simulink model "sdbe_11_11"  (R2012b)
settings: Solver=VariableStepDiscrete  SolverMode=SingleTasking  StartTime=0.0  StopTime=10000  RelTol=1e-3
PreLoadFcn:
  | counter_vals
undefined symbols (not defined in the file or in its folder): sfp
libraries: xbsIndex_r4 x9223, casper_library_misc x39, casper_library_delays x27, dspsigops x16, xps_library x10, r2dbe_vdif_lib x4, r2dbe_adc_lib x3, simulink x1
(part 61 of 78)

== system sdbe_11_11/vdif_2/hdr/w2 ==
  note: 3 bits
  note: According to VDIF documentation for W2
      |
      |
      | bit 31-29 (3): VDIF version number
      | In ALMA EDV it is 0
      |
      | bits 28-24: log2(nchans)
      | 1 channel, so this will be 0
      |
      | bits 23-0: Data Frame length in units
      | of 8 bytes
      | Each 64 bit word is 8 bytes, so 1024 of these
  note: data_fram_length_in_8 byte words
  note: V3
  note: 5 bits
  note: log2(nchans) = 0
  Constant : xbsIndex_r4/Constant  const=0  gui_display_data_type=Fixed-point  arith_type=Unsigned  n_bits=3  bin_pt=0  preci_type=Single  exp_width=8  frac_width=24  explicit_period=on  period=1  equ=P=C  opselect=C  inp2=PCIN>>17  opr=+  inp1=P  carry=CIN  dbl_ovrd=off  block_type=constant
  Constant1 : xbsIndex_r4/Constant  const=3  gui_display_data_type=Fixed-point  arith_type=Unsigned  n_bits=5  bin_pt=0  preci_type=Single  exp_width=8  frac_width=24  explicit_period=on  period=1  equ=P=C  opselect=C  inp2=PCIN>>17  opr=+  inp1=P  carry=CIN  dbl_ovrd=off  block_type=constant
  Constant2 : xbsIndex_r4/Constant  const=132  gui_display_data_type=Fixed-point  arith_type=Unsigned  n_bits=24  bin_pt=0  preci_type=Single  exp_width=8  frac_width=24  explicit_period=on  period=1  equ=P=C  opselect=C  inp2=PCIN>>17  opr=+  inp1=P  carry=CIN  dbl_ovrd=off  block_type=constant
  Convert1 : xbsIndex_r4/Convert  gui_display_data_type=Fixed-point  arith_type=Unsigned  n_bits=32  bin_pt=0  float_type=Single  exp_bits=8  fraction_bits=24  quantization=Truncate  overflow=Wrap  en=off  latency=0  dbl_ovrd=off  pipeline=off  block_type=convert
  Terminator : Terminator
  bus_create : Subsystem  mask(bus_create){inputNum=3}
      mask prompts: inputNum "Number of inputs:"
      mask init:
      | bus_create_init(gcb,...
      |     'inputNum', inputNum);
  frame_len : Subsystem  Tag=xps:sw_reg  AncestorBlock=xps_library/software register  mask(swreg){mode=one value, io_dir=To Processor, io_delay=0, sample_period=1, names=reg, bitwidths=32, arith_types=0, bin_pts=0, sim_port=on, show_format=off}
      mask prompts: io_dir "I/O direction"; io_delay "I/O delay"; sample_period "Sample period"; names "Name:"; bitwidths "Bitwidth:"; arith_types "Type (ufix=0, fix=1, bool=2):"; bin_pts "Binary pt:"; sim_port "Provide sim input/output?"; show_format "Print format string?"
      mask init:
      | swreg_init(gcb)
      settings: AttributesFormatString=1output
      mask TypeOptions mode: one value | fields of equal size | fields of arbitrary size
      mask Callback mode: swreg_cb(gcb);
      mask TypeOptions io_dir: To Processor | From Processor
      mask Callback io_dir:
      | mask_enables = get_param(gcb, 'MaskEnables');
      | mask_names = get_param(gcb, 'MaskNames');
      | if strcmp(get_param(gcb, 'io_dir'), 'To Processor'),
      |     mask_enables{ismember(mask_names, 'sample_period')} = 'off';
      | else
      |     mask_enables{ismember(mask_names, 'sample_period')} = 'on';
      | end
      | set_param(gcb, 'MaskEnables', mask_enables);
      mask Callback bitwidths:
      | swreg_maskcheck(gcb);
      | % blk = gcb;
      | % mode = get_param(blk, 'mode');
      | % current_widths = eval(get_param(blk, 'bitwidths'));
      | % if (strcmp(mode, 'one value') || strcmp(mode, 'fields of equal size')) && (length(current_widths) > 1),
      | %     error('Only one width may be specified for this mode.');
      | % elseif strcmp(mode, 'fields of arbitrary size')
      | %     current_names = textscan(strtrim(strrep(strrep(get_param(blk, 'names'), ']', ''), '[', '')), '%s');
      | %     current_names = current_names{1};
      | %     numios = length(current_names);
      | %     if length(current_widths) ~= numios,
      | %         error('%d field names specified, but %d widths?', numios, length(current_widths));
      | %     end
      | % end
      | % total_width = 0;
      | % for ctr = 1 : length(current_widths),
      | %     total_width = total_width + current_widths(ctr);
      | % end
      | % if total_width > 32,
      | %     error('Total width must be 32 or less, set to %d.', total_width);
      | % end
      mask Callback arith_types:
      | [numios, ~, ~, ~, current_types] = swreg_maskcheck(gcb);
      | % blk = gcb;
      | % mode = get_param(blk, 'mode');
      | % current_types = eval(get_param(blk, 'arith_types'));
      | % numios = length(current_types);
      | % if (strcmp(mode, 'one value') || strcmp(mode, 'fields of equal size')) && (length(current_types) > 1),
      | %     error('Only one type may be specified for this mode.');
      | % elseif strcmp(mode, 'fields of arbitrary size')
      | %     current_names = textscan(strtrim(strrep(strrep(get_param(blk, 'names'), ']', ''), '[', '')), '%s');
      | %     current_names = current_names{1};
      | %     numios = length(current_names);
      | %     if length(current_types) ~= numios,
      | %         error('%d field names specified, but %d types?', numios, length(current_types));
      | %     end
      | % end
      | problem = 0;
      | for ctr = 1 : numios,
      |     t = current_types(ctr);
      |     if (t < 0) || (t > 2),
      |         problem = t;
      |         ctr = numios + 1;
      |     end
      | end
      | if problem ~= 0,
      |     error('Type cannot be %i, must be 0, 1 or 2.', problem);
      | end
      mask Callback bin_pts:
      | swreg_maskcheck(gcb);
      | % blk = gcb;
      | % mode = get_param(blk, 'mode');
      | % current_bins = eval(get_param(blk, 'bin_pts'));
      | % if (strcmp(mode, 'one value') || strcmp(mode, 'fields of equal size')) && (length(current_bins) > 1),
      | %     error('Only one binary pt may be specified for this mode.');
      | % elseif strcmp(mode, 'fields of arbitrary size')
      | %     current_names = textscan(strtrim(strrep(strrep(get_param(blk, 'names'), ']', ''), '[', '')), '%s');
      | %     current_names = current_names{1};
      | %     numios = length(current_names);
      | %     if length(current_bins) ~= numios,
      | %         error('%d field names specified, but %d binary pts?', numios, length(current_bins));
      | %     end
      | % end
  w2 : Outport
  wires:
  Constant1/1 -> bus_create/2(in2)
  bus_create/1(bus_out) -> w2/1
  Constant/1 -> bus_create/1(in1)
  Constant2/1 -> Convert1/1, bus_create/3(in3)
  frame_len/1(sim_out) -> Terminator/1
  Convert1/1 -> frame_len/1(out_reg)

== system sdbe_11_11/vdif_2/hdr/w3 ==
  note: 1 bits
  note: 16 bits
  note: 10 bits
  note: bits per samp minus 1
  note: 5 bits
  note: real_or_comp
  note: According to VDIF documentation for W3
      |
      |
      | bit 31: Real Data or Complex
      | 0 for real data
      |
      | bits 30-26 #bits/sample -1
      | 2 bits per sample -1 =1
      |
      | bits 25-16: thread ID (0 to 1023)
      | not multi-threaded, so just 0
      |
      | Bits 15-0: station ID
  Constant : xbsIndex_r4/Constant  const=1  gui_display_data_type=Fixed-point  arith_type=Unsigned  n_bits=1  bin_pt=0  preci_type=Single  exp_width=8  frac_width=24  explicit_period=on  period=1  equ=P=C  opselect=C  inp2=PCIN>>17  opr=+  inp1=P  carry=CIN  dbl_ovrd=off  block_type=constant
  Constant1 : xbsIndex_r4/Constant  const=1  gui_display_data_type=Fixed-point  arith_type=Unsigned  n_bits=5  bin_pt=0  preci_type=Single  exp_width=8  frac_width=24  explicit_period=on  period=1  equ=P=C  opselect=C  inp2=PCIN>>17  opr=+  inp1=P  carry=CIN  dbl_ovrd=off  block_type=constant
  Constant2 : Constant  Value=1023
  Constant3 : Constant  Value=3097
  Slice : xbsIndex_r4/Slice  nbits=16  boolean_output=off  mode=Lower Bit Location + Width  bit1=0  base1=MSB of Input  bit0=0  base0=LSB of Input  dbl_ovrd=off  block_type=slice
  Slice1 : xbsIndex_r4/Slice  nbits=10  boolean_output=off  mode=Lower Bit Location + Width  bit1=0  base1=MSB of Input  bit0=0  base0=LSB of Input  dbl_ovrd=off  block_type=slice
  bus_create3 : Subsystem  mask(bus_create){inputNum=4}
      mask prompts: inputNum "Number of inputs:"
      mask init:
      | bus_create_init(gcb,...
      |     'inputNum', inputNum);
  pipeline : casper_library_delays/pipeline  latency=1
      settings: AttributesFormatString=Latency = %<latency>
  pipeline1 : casper_library_delays/pipeline  latency=1
      settings: AttributesFormatString=Latency = %<latency>
  station_id : Subsystem  Tag=xps:sw_reg  AncestorBlock=xps_library/software register  mask(swreg){mode=one value, io_dir=From Processor, io_delay=0, sample_period=1, names=reg, bitwidths=32, arith_types=0, bin_pts=0, sim_port=on, show_format=off}
      mask prompts: io_dir "I/O direction"; io_delay "I/O delay"; sample_period "Sample period"; names "Name:"; bitwidths "Bitwidth:"; arith_types "Type (ufix=0, fix=1, bool=2):"; bin_pts "Binary pt:"; sim_port "Provide sim input/output?"; show_format "Print format string?"
      mask init:
      | swreg_init(gcb)
      settings: AttributesFormatString=1input
      mask TypeOptions mode: one value | fields of equal size | fields of arbitrary size
      mask Callback mode: swreg_cb(gcb);
      mask TypeOptions io_dir: To Processor | From Processor
      mask Callback io_dir:
      | mask_enables = get_param(gcb, 'MaskEnables');
      | mask_names = get_param(gcb, 'MaskNames');
      | if strcmp(get_param(gcb, 'io_dir'), 'To Processor'),
      |     mask_enables{ismember(mask_names, 'sample_period')} = 'off';
      | else
      |     mask_enables{ismember(mask_names, 'sample_period')} = 'on';
      | end
      | set_param(gcb, 'MaskEnables', mask_enables);
      mask Callback bitwidths:
      | swreg_maskcheck(gcb);
      | % blk = gcb;
      | % mode = get_param(blk, 'mode');
      | % current_widths = eval(get_param(blk, 'bitwidths'));
      | % if (strcmp(mode, 'one value') || strcmp(mode, 'fields of equal size')) && (length(current_widths) > 1),
      | %     error('Only one width may be specified for this mode.');
      | % elseif strcmp(mode, 'fields of arbitrary size')
      | %     current_names = textscan(strtrim(strrep(strrep(get_param(blk, 'names'), ']', ''), '[', '')), '%s');
      | %     current_names = current_names{1};
      | %     numios = length(current_names);
      | %     if length(current_widths) ~= numios,
      | %         error('%d field names specified, but %d widths?', numios, length(current_widths));
      | %     end
      | % end
      | % total_width = 0;
      | % for ctr = 1 : length(current_widths),
      | %     total_width = total_width + current_widths(ctr);
      | % end
      | % if total_width > 32,
      | %     error('Total width must be 32 or less, set to %d.', total_width);
      | % end
      mask Callback arith_types:
      | [numios, ~, ~, ~, current_types] = swreg_maskcheck(gcb);
      | % blk = gcb;
      | % mode = get_param(blk, 'mode');
      | % current_types = eval(get_param(blk, 'arith_types'));
      | % numios = length(current_types);
      | % if (strcmp(mode, 'one value') || strcmp(mode, 'fields of equal size')) && (length(current_types) > 1),
      | %     error('Only one type may be specified for this mode.');
      | % elseif strcmp(mode, 'fields of arbitrary size')
      | %     current_names = textscan(strtrim(strrep(strrep(get_param(blk, 'names'), ']', ''), '[', '')), '%s');
      | %     current_names = current_names{1};
      | %     numios = length(current_names);
      | %     if length(current_types) ~= numios,
      | %         error('%d field names specified, but %d types?', numios, length(current_types));
      | %     end
      | % end
      | problem = 0;
      | for ctr = 1 : numios,
      |     t = current_types(ctr);
      |     if (t < 0) || (t > 2),
      |         problem = t;
      |         ctr = numios + 1;
      |     end
      | end
      | if problem ~= 0,
      |     error('Type cannot be %i, must be 0, 1 or 2.', problem);
      | end
      mask Callback bin_pts:
      | swreg_maskcheck(gcb);
      | % blk = gcb;
      | % mode = get_param(blk, 'mode');
      | % current_bins = eval(get_param(blk, 'bin_pts'));
      | % if (strcmp(mode, 'one value') || strcmp(mode, 'fields of equal size')) && (length(current_bins) > 1),
      | %     error('Only one binary pt may be specified for this mode.');
      | % elseif strcmp(mode, 'fields of arbitrary size')
      | %     current_names = textscan(strtrim(strrep(strrep(get_param(blk, 'names'), ']', ''), '[', '')), '%s');
      | %     current_names = current_names{1};
      | %     numios = length(current_names);
      | %     if length(current_bins) ~= numios,
      | %         error('%d field names specified, but %d binary pts?', numios, length(current_bins));
      | %     end
      | % end
  thread_id : Subsystem  Tag=xps:sw_reg  AncestorBlock=xps_library/software register  mask(swreg){mode=one value, io_dir=From Processor, io_delay=0, sample_period=1, names=reg, bitwidths=32, arith_types=0, bin_pts=0, sim_port=on, show_format=off}
      mask prompts: io_dir "I/O direction"; io_delay "I/O delay"; sample_period "Sample period"; names "Name:"; bitwidths "Bitwidth:"; arith_types "Type (ufix=0, fix=1, bool=2):"; bin_pts "Binary pt:"; sim_port "Provide sim input/output?"; show_format "Print format string?"
      mask init:
      | swreg_init(gcb)
      settings: AttributesFormatString=1input
      mask TypeOptions mode: one value | fields of equal size | fields of arbitrary size
      mask Callback mode: swreg_cb(gcb);
      mask TypeOptions io_dir: To Processor | From Processor
      mask Callback io_dir:
      | mask_enables = get_param(gcb, 'MaskEnables');
      | mask_names = get_param(gcb, 'MaskNames');
      | if strcmp(get_param(gcb, 'io_dir'), 'To Processor'),
      |     mask_enables{ismember(mask_names, 'sample_period')} = 'off';
      | else
      |     mask_enables{ismember(mask_names, 'sample_period')} = 'on';
      | end
      | set_param(gcb, 'MaskEnables', mask_enables);
      mask Callback bitwidths:
      | swreg_maskcheck(gcb);
      | % blk = gcb;
      | % mode = get_param(blk, 'mode');
      | % current_widths = eval(get_param(blk, 'bitwidths'));
      | % if (strcmp(mode, 'one value') || strcmp(mode, 'fields of equal size')) && (length(current_widths) > 1),
      | %     error('Only one width may be specified for this mode.');
      | % elseif strcmp(mode, 'fields of arbitrary size')
      | %     current_names = textscan(strtrim(strrep(strrep(get_param(blk, 'names'), ']', ''), '[', '')), '%s');
      | %     current_names = current_names{1};
      | %     numios = length(current_names);
      | %     if length(current_widths) ~= numios,
      | %         error('%d field names specified, but %d widths?', numios, length(current_widths));
      | %     end
      | % end
      | % total_width = 0;
      | % for ctr = 1 : length(current_widths),
      | %     total_width = total_width + current_widths(ctr);
      | % end
      | % if total_width > 32,
      | %     error('Total width must be 32 or less, set to %d.', total_width);
      | % end
      mask Callback arith_types:
      | [numios, ~, ~, ~, current_types] = swreg_maskcheck(gcb);
      | % blk = gcb;
      | % mode = get_param(blk, 'mode');
      | % current_types = eval(get_param(blk, 'arith_types'));
      | % numios = length(current_types);
      | % if (strcmp(mode, 'one value') || strcmp(mode, 'fields of equal size')) && (length(current_types) > 1),
      | %     error('Only one type may be specified for this mode.');
      | % elseif strcmp(mode, 'fields of arbitrary size')
      | %     current_names = textscan(strtrim(strrep(strrep(get_param(blk, 'names'), ']', ''), '[', '')), '%s');
      | %     current_names = current_names{1};
      | %     numios = length(current_names);
      | %     if length(current_types) ~= numios,
      | %         error('%d field names specified, but %d types?', numios, length(current_types));
      | %     end
      | % end
      | problem = 0;
      | for ctr = 1 : numios,
      |     t = current_types(ctr);
      |     if (t < 0) || (t > 2),
      |         problem = t;
      |         ctr = numios + 1;
      |     end
      | end
      | if problem ~= 0,
      |     error('Type cannot be %i, must be 0, 1 or 2.', problem);
      | end
      mask Callback bin_pts:
      | swreg_maskcheck(gcb);
      | % blk = gcb;
      | % mode = get_param(blk, 'mode');
      | % current_bins = eval(get_param(blk, 'bin_pts'));
      | % if (strcmp(mode, 'one value') || strcmp(mode, 'fields of equal size')) && (length(current_bins) > 1),
      | %     error('Only one binary pt may be specified for this mode.');
      | % elseif strcmp(mode, 'fields of arbitrary size')
      | %     current_names = textscan(strtrim(strrep(strrep(get_param(blk, 'names'), ']', ''), '[', '')), '%s');
      | %     current_names = current_names{1};
      | %     numios = length(current_names);
      | %     if length(current_bins) ~= numios,
      | %         error('%d field names specified, but %d binary pts?', numios, length(current_bins));
      | %     end
      | % end
  w3 : Outport
  wires:
  pipeline1/1 -> Slice/1
  pipeline/1 -> Slice1/1
  Slice/1 -> bus_create3/4(in4)
  Constant/1 -> bus_create3/1(in1)
  Slice1/1 -> bus_create3/3(in3)
  Constant1/1 -> bus_create3/2(in2)
  thread_id/1(in_reg) -> pipeline/1
  Constant2/1 -> thread_id/1(sim_1)
  Constant3/1 -> station_id/1(sim_1)
  station_id/1(in_reg) -> pipeline1/1
  bus_create3/1(bus_out) -> w3/1

== system sdbe_11_11/vdif_2/hdr/w6_w7 ==
  note: in simulation because I don't have the fixed point tool kit,
      | the 64 bit counter is messing up so I am getting values starting with 1 rather than 0
      | I think in compile this will work
  note: start this at 2^64-1, so its the last value of the counter,
      | then when enabled the first value will be 0
  note: According to VDIF documentation for W5
      | and EDV doc for ALMA
      |
      | not sure what the packet serial number is,
      | apparently it is appended in front of the packet
      | for transfer, but im not sure where it comes from
      |
      | This uses UDP, so I wonder when it is appended
      |
      | Right now I have a software register in there as a place holder
  note: word 7 is MOst sig 32
  note: word 6 is Least sig
  start_of_frame : Inport
  Convert1 : xbsIndex_r4/Convert  gui_display_data_type=Fixed-point  arith_type=Unsigned  n_bits=32  bin_pt=0  float_type=Single  exp_bits=8  fraction_bits=24  quantization=Truncate  overflow=Wrap  en=off  latency=0  dbl_ovrd=off  pipeline=off  block_type=convert
  Convert2 : xbsIndex_r4/Convert  gui_display_data_type=Fixed-point  arith_type=Unsigned  n_bits=32  bin_pt=0  float_type=Single  exp_bits=8  fraction_bits=24  quantization=Truncate  overflow=Wrap  en=off  latency=0  dbl_ovrd=off  pipeline=off  block_type=convert
  Counter : xbsIndex_r4/Counter  cnt_type=Free Running  cnt_to=Inf  operation=Up  start_count=2^64-1  cnt_by_val=1  arith_type=Unsigned  n_bits=64  bin_pt=0  load_pin=off  rst=off  en=on  explicit_period=on  period=1  dbl_ovrd=off  use_behavioral_HDL=off  implementation=Fabric  block_type=counter
  Delay : xbsIndex_r4/Delay  rst=off  infoeditControl=Selection of Reset will increase slice count due to use of real FFs and instead of SRLs  en=off  latency=1  dbl_ovrd=off  reg_retiming=off  block_type=delay
  Delay1 : xbsIndex_r4/Delay  rst=off  infoeditControl=Selection of Reset will increase slice count due to use of real FFs and instead of SRLs  en=off  latency=1  dbl_ovrd=off  reg_retiming=off  block_type=delay
  Terminator : Terminator
  Terminator1 : Terminator
  lower_32 : xbsIndex_r4/Slice  nbits=32  boolean_output=off  mode=Lower Bit Location + Width  bit1=0  base1=LSB of Input  bit0=0  base0=LSB of Input  dbl_ovrd=off  block_type=slice
  psn_high : Subsystem  Tag=xps:sw_reg  AncestorBlock=xps_library/software register  mask(swreg){mode=one value, io_dir=To Processor, io_delay=0, sample_period=1, names=reg, bitwidths=32, arith_types=0, bin_pts=0, sim_port=on, show_format=off}
      mask prompts: io_dir "I/O direction"; io_delay "I/O delay"; sample_period "Sample period"; names "Name:"; bitwidths "Bitwidth:"; arith_types "Type (ufix=0, fix=1, bool=2):"; bin_pts "Binary pt:"; sim_port "Provide sim input/output?"; show_format "Print format string?"
      mask init:
      | swreg_init(gcb)
      settings: AttributesFormatString=1output
      mask TypeOptions mode: one value | fields of equal size | fields of arbitrary size
      mask Callback mode: swreg_cb(gcb);
      mask TypeOptions io_dir: To Processor | From Processor
      mask Callback io_dir:
      | mask_enables = get_param(gcb, 'MaskEnables');
      | mask_names = get_param(gcb, 'MaskNames');
      | if strcmp(get_param(gcb, 'io_dir'), 'To Processor'),
      |     mask_enables{ismember(mask_names, 'sample_period')} = 'off';
      | else
      |     mask_enables{ismember(mask_names, 'sample_period')} = 'on';
      | end
      | set_param(gcb, 'MaskEnables', mask_enables);
      mask Callback bitwidths:
      | swreg_maskcheck(gcb);
      | % blk = gcb;
      | % mode = get_param(blk, 'mode');
      | % current_widths = eval(get_param(blk, 'bitwidths'));
      | % if (strcmp(mode, 'one value') || strcmp(mode, 'fields of equal size')) && (length(current_widths) > 1),
      | %     error('Only one width may be specified for this mode.');
      | % elseif strcmp(mode, 'fields of arbitrary size')
      | %     current_names = textscan(strtrim(strrep(strrep(get_param(blk, 'names'), ']', ''), '[', '')), '%s');
      | %     current_names = current_names{1};
      | %     numios = length(current_names);
      | %     if length(current_widths) ~= numios,
      | %         error('%d field names specified, but %d widths?', numios, length(current_widths));
      | %     end
      | % end
      | % total_width = 0;
      | % for ctr = 1 : length(current_widths),
      | %     total_width = total_width + current_widths(ctr);
      | % end
      | % if total_width > 32,
      | %     error('Total width must be 32 or less, set to %d.', total_width);
      | % end
      mask Callback arith_types:
      | [numios, ~, ~, ~, current_types] = swreg_maskcheck(gcb);
      | % blk = gcb;
      | % mode = get_param(blk, 'mode');
      | % current_types = eval(get_param(blk, 'arith_types'));
      | % numios = length(current_types);
      | % if (strcmp(mode, 'one value') || strcmp(mode, 'fields of equal size')) && (length(current_types) > 1),
      | %     error('Only one type may be specified for this mode.');
      | % elseif strcmp(mode, 'fields of arbitrary size')
      | %     current_names = textscan(strtrim(strrep(strrep(get_param(blk, 'names'), ']', ''), '[', '')), '%s');
      | %     current_names = current_names{1};
      | %     numios = length(current_names);
      | %     if length(current_types) ~= numios,
      | %         error('%d field names specified, but %d types?', numios, length(current_types));
      | %     end
      | % end
      | problem = 0;
      | for ctr = 1 : numios,
      |     t = current_types(ctr);
      |     if (t < 0) || (t > 2),
      |         problem = t;
      |         ctr = numios + 1;
      |     end
      | end
      | if problem ~= 0,
      |     error('Type cannot be %i, must be 0, 1 or 2.', problem);
      | end
      mask Callback bin_pts:
      | swreg_maskcheck(gcb);
      | % blk = gcb;
      | % mode = get_param(blk, 'mode');
      | % current_bins = eval(get_param(blk, 'bin_pts'));
      | % if (strcmp(mode, 'one value') || strcmp(mode, 'fields of equal size')) && (length(current_bins) > 1),
      | %     error('Only one binary pt may be specified for this mode.');
      | % elseif strcmp(mode, 'fields of arbitrary size')
      | %     current_names = textscan(strtrim(strrep(strrep(get_param(blk, 'names'), ']', ''), '[', '')), '%s');
      | %     current_names = current_names{1};
      | %     numios = length(current_names);
      | %     if length(current_bins) ~= numios,
      | %         error('%d field names specified, but %d binary pts?', numios, length(current_bins));
      | %     end
      | % end
  psn_low : Subsystem  Tag=xps:sw_reg  AncestorBlock=xps_library/software register  mask(swreg){mode=one value, io_dir=To Processor, io_delay=0, sample_period=1, names=reg, bitwidths=32, arith_types=0, bin_pts=0, sim_port=on, show_format=off}
      mask prompts: io_dir "I/O direction"; io_delay "I/O delay"; sample_period "Sample period"; names "Name:"; bitwidths "Bitwidth:"; arith_types "Type (ufix=0, fix=1, bool=2):"; bin_pts "Binary pt:"; sim_port "Provide sim input/output?"; show_format "Print format string?"
      mask init:
      | swreg_init(gcb)
      settings: AttributesFormatString=1output
      mask TypeOptions mode: one value | fields of equal size | fields of arbitrary size
      mask Callback mode: swreg_cb(gcb);
      mask TypeOptions io_dir: To Processor | From Processor
      mask Callback io_dir:
      | mask_enables = get_param(gcb, 'MaskEnables');
      | mask_names = get_param(gcb, 'MaskNames');
      | if strcmp(get_param(gcb, 'io_dir'), 'To Processor'),
      |     mask_enables{ismember(mask_names, 'sample_period')} = 'off';
      | else
      |     mask_enables{ismember(mask_names, 'sample_period')} = 'on';
      | end
      | set_param(gcb, 'MaskEnables', mask_enables);
      mask Callback bitwidths:
      | swreg_maskcheck(gcb);
      | % blk = gcb;
      | % mode = get_param(blk, 'mode');
      | % current_widths = eval(get_param(blk, 'bitwidths'));
      | % if (strcmp(mode, 'one value') || strcmp(mode, 'fields of equal size')) && (length(current_widths) > 1),
      | %     error('Only one width may be specified for this mode.');
      | % elseif strcmp(mode, 'fields of arbitrary size')
      | %     current_names = textscan(strtrim(strrep(strrep(get_param(blk, 'names'), ']', ''), '[', '')), '%s');
      | %     current_names = current_names{1};
      | %     numios = length(current_names);
      | %     if length(current_widths) ~= numios,
      | %         error('%d field names specified, but %d widths?', numios, length(current_widths));
      | %     end
      | % end
      | % total_width = 0;
      | % for ctr = 1 : length(current_widths),
      | %     total_width = total_width + current_widths(ctr);
      | % end
      | % if total_width > 32,
      | %     error('Total width must be 32 or less, set to %d.', total_width);
      | % end
      mask Callback arith_types:
      | [numios, ~, ~, ~, current_types] = swreg_maskcheck(gcb);
      | % blk = gcb;
      | % mode = get_param(blk, 'mode');
      | % current_types = eval(get_param(blk, 'arith_types'));
      | % numios = length(current_types);
      | % if (strcmp(mode, 'one value') || strcmp(mode, 'fields of equal size')) && (length(current_types) > 1),
      | %     error('Only one type may be specified for this mode.');
      | % elseif strcmp(mode, 'fields of arbitrary size')
      | %     current_names = textscan(strtrim(strrep(strrep(get_param(blk, 'names'), ']', ''), '[', '')), '%s');
      | %     current_names = current_names{1};
      | %     numios = length(current_names);
      | %     if length(current_types) ~= numios,
      | %         error('%d field names specified, but %d types?', numios, length(current_types));
      | %     end
      | % end
      | problem = 0;
      | for ctr = 1 : numios,
      |     t = current_types(ctr);
      |     if (t < 0) || (t > 2),
      |         problem = t;
      |         ctr = numios + 1;
      |     end
      | end
      | if problem ~= 0,
      |     error('Type cannot be %i, must be 0, 1 or 2.', problem);
      | end
      mask Callback bin_pts:
      | swreg_maskcheck(gcb);
      | % blk = gcb;
      | % mode = get_param(blk, 'mode');
      | % current_bins = eval(get_param(blk, 'bin_pts'));
      | % if (strcmp(mode, 'one value') || strcmp(mode, 'fields of equal size')) && (length(current_bins) > 1),
      | %     error('Only one binary pt may be specified for this mode.');
      | % elseif strcmp(mode, 'fields of arbitrary size')
      | %     current_names = textscan(strtrim(strrep(strrep(get_param(blk, 'names'), ']', ''), '[', '')), '%s');
      | %     current_names = current_names{1};
      | %     numios = length(current_names);
      | %     if length(current_bins) ~= numios,
      | %         error('%d field names specified, but %d binary pts?', numios, length(current_bins));
      | %     end
      | % end
  upper_32 : xbsIndex_r4/Slice  nbits=32  boolean_output=off  mode=Lower Bit Location + Width  bit1=0  base1=MSB of Input  bit0=32  base0=LSB of Input  dbl_ovrd=off  block_type=slice
  w6 : Outport
  w7 : Outport  Port=2
  wires:
  start_of_frame/1 -> Counter/1
  upper_32/1 -> Convert2/1, Delay/1
  lower_32/1 -> Convert1/1, Delay1/1
  Counter/1 -> lower_32/1, upper_32/1
  psn_low/1(sim_out) -> Terminator/1
  Convert1/1 -> psn_low/1(out_reg)
  psn_high/1(sim_out) -> Terminator1/1
  Convert2/1 -> psn_high/1(out_reg)
  Delay/1 -> w7/1
  Delay1/1 -> w6/1

== system sdbe_11_11/vdif_2/hdr_to_scope1/diagnose_beng_hdr ==
  tx_data : Inport
  tx_val : Inport  Port=2
  Disregard Subsystem : xbsIndex_r4/Disregard Subsystem  Tag=discardX  block_type=disregard
  Scope : Scope  NumInputPorts=2
      settings: TimeRange=1.649420126233963  YMin=-1~-1  YMax=1~1
  wires:
  tx_data/1 -> Scope/1  "data"
  tx_val/1 -> Scope/2  "vals"

== system sdbe_11_11/vdif_2/hdr_to_scope3/beng_w45 ==
  note: VTP so need to wait one more clock
  data : Inport
  val : Inport  Port=2
  spec_val : Inport  Port=3
  Constant : xbsIndex_r4/Constant  const=0  gui_display_data_type=Fixed-point  arith_type=Unsigned  n_bits=64  bin_pt=0  preci_type=Single  exp_width=8  frac_width=24  explicit_period=on  period=1  equ=P=C  opselect=C  inp2=PCIN>>17  opr=+  inp1=P  carry=CIN  dbl_ovrd=off  block_type=constant
  Disregard Subsystem : xbsIndex_r4/Disregard Subsystem  Tag=discardX  block_type=disregard
  Gateway Out{,1..4} (5 alike) : xbsIndex_r4/Gateway Out  inherit_from_input=off  hdl_port=on  timing_constraint=None  locs_specified=off  LOCs={}  UseAsDAC=off  DACChannel='1'  block_type=gatewayout
  Mux : xbsIndex_r4/Mux  inputs=2  en=off  latency=0  precision=Full  arith_type=Unsigned  n_bits=16  bin_pt=14  quantization=Truncate  overflow=Wrap  dbl_ovrd=off  block_type=mux
  Mux1 : Mux  Inputs=2
  Mux2 : Mux  Inputs=3
  Scope : Scope  NumInputPorts=2
      settings: TimeRange=1.649420126233963  YMin=-1~-1  YMax=1~1  SaveName=ScopeData14
  beng_hdr_from_data : Subsystem
  wires:
  val/1 -> Gateway Out3/1
  Gateway Out2/1 -> Mux2/3
  Gateway Out/1 -> Mux2/1
  Constant/1 -> Mux/2
  Mux/1 -> beng_hdr_from_data/1(hdr_64)
  [val_45] -> Mux/1
  Mux1/1 -> Scope/2  "val_yellow__w45_val_pink"
  Gateway Out1/1 -> Mux2/2
  beng_hdr_from_data/3(fcount) -> Gateway Out2/1
  Gateway Out3/1 -> Mux1/1
  Gateway Out4/1 -> Mux1/2
  data/1 -> Mux/3
  beng_hdr_from_data/2(bcount) -> Gateway Out1/1
  beng_hdr_from_data/1(ccount) -> Gateway Out/1
  spec_val/1 -> Gateway Out4/1, [val_45]
  Mux2/1 -> Scope/1  "c_yellow__b_pink__f_blue"

== system sdbe_11_11/vdif_2/hdr_to_scope3/data_p0r ==
  note: VTP so need to wait one more clock
  data : Inport
  val : Inport  Port=2
  spec_val : Inport  Port=3
  Constant : xbsIndex_r4/Constant  const=0  gui_display_data_type=Fixed-point  arith_type=Unsigned  n_bits=64  bin_pt=0  preci_type=Single  exp_width=8  frac_width=24  explicit_period=on  period=1  equ=P=C  opselect=C  inp2=PCIN>>17  opr=+  inp1=P  carry=CIN  dbl_ovrd=off  block_type=constant
  Disregard Subsystem : xbsIndex_r4/Disregard Subsystem  Tag=discardX  block_type=disregard
  Gateway Out{1..40} (40 alike) : xbsIndex_r4/Gateway Out  inherit_from_input=off  hdl_port=on  timing_constraint=None  locs_specified=off  LOCs={}  UseAsDAC=off  DACChannel='1'  block_type=gatewayout
  Mux : xbsIndex_r4/Mux  inputs=2  en=off  latency=0  precision=Full  arith_type=Unsigned  n_bits=16  bin_pt=14  quantization=Truncate  overflow=Wrap  dbl_ovrd=off  block_type=mux
  Mux{1,3,5,7} (4 alike) : Mux  Inputs=2
  Mux{2,4,6,8} (4 alike) : Mux  Inputs=8
  Scope{,1..3} (4 alike) : Scope  NumInputPorts=2
      Scope settings: TimeRange=1.649420126233963  YMin=-1~-1  YMax=1~1  SaveName=ScopeData12
      Scope1 settings: TimeRange=1.649420126233963  YMin=-1~-1  YMax=1~1  SaveName=ScopeData18
      Scope2 settings: TimeRange=1.649420126233963  YMin=-1~-1  YMax=1~1  SaveName=ScopeData19
      Scope3 settings: TimeRange=1.649420126233963  YMin=-1~-1  YMax=1~1  SaveName=ScopeData20
  Subsystem : Subsystem
  bus_expand : Subsystem  AncestorBlock=casper_library_flow_control/bus_expand  mask(bus_expand){mode=divisions of equal size, outputNum=8, outputWidth=2, outputBinaryPt=0, outputArithmeticType=0, show_format=off, outputToWorkspace=off, variablePrefix=out, outputToModelAsWell=on}
      mask prompts: outputNum "Number of outputs:"; outputWidth "Output width:"; outputBinaryPt "Output binary point position:"; outputArithmeticType "Output arithmetic type (ufix=0, fix=1, bool=2):"; show_format "Print format string?"; outputToWorkspace "Output to workspace?"; variablePrefix "Variable name prefix:"; outputToModelAsWell "Output to model as well?"
      mask help:
      | Expands a 'bus' made using a bus_create or Xilinx
      | concat block.
      | The input will be divided into the specified number
      | of outputs with the specified arithmetic types.
      | Divisions are made from most significant bit.
      mask init: same as sdbe_11_11/get_data_from_pkt/scope/bus_expand1
      settings: AttributesFormatString=8 outputs
      mask TypeOptions mode: divisions of equal size | divisions of arbitrary size
      mask Callback mode: bus_expand_callback();
      mask Callback outputWidth: bus_expand_callback();
      mask Callback outputToWorkspace: bus_expand_callback();
  bus_expand1 : Subsystem  AncestorBlock=casper_library_flow_control/bus_expand  mask(bus_expand){mode=divisions of equal size, outputNum=8, outputWidth=2, outputBinaryPt=0, outputArithmeticType=0, show_format=off, outputToWorkspace=off, variablePrefix=out, outputToModelAsWell=on}
      mask prompts: outputNum "Number of outputs:"; outputWidth "Output width:"; outputBinaryPt "Output binary point position:"; outputArithmeticType "Output arithmetic type (ufix=0, fix=1, bool=2):"; show_format "Print format string?"; outputToWorkspace "Output to workspace?"; variablePrefix "Variable name prefix:"; outputToModelAsWell "Output to model as well?"
      mask help:
      | Expands a 'bus' made using a bus_create or Xilinx
      | concat block.
      | The input will be divided into the specified number
      | of outputs with the specified arithmetic types.
      | Divisions are made from most significant bit.
      mask init: same as sdbe_11_11/get_data_from_pkt/scope/bus_expand1
      settings: AttributesFormatString=8 outputs
      mask TypeOptions mode: divisions of equal size | divisions of arbitrary size
      mask Callback mode: bus_expand_callback();
      mask Callback outputWidth: bus_expand_callback();
      mask Callback outputToWorkspace: bus_expand_callback();
  bus_expand2 : Subsystem  AncestorBlock=casper_library_flow_control/bus_expand  mask(bus_expand){mode=divisions of equal size, outputNum=8, outputWidth=2, outputBinaryPt=0, outputArithmeticType=0, show_format=off, outputToWorkspace=off, variablePrefix=out, outputToModelAsWell=on}
      mask prompts: outputNum "Number of outputs:"; outputWidth "Output width:"; outputBinaryPt "Output binary point position:"; outputArithmeticType "Output arithmetic type (ufix=0, fix=1, bool=2):"; show_format "Print format string?"; outputToWorkspace "Output to workspace?"; variablePrefix "Variable name prefix:"; outputToModelAsWell "Output to model as well?"
      mask help:
      | Expands a 'bus' made using a bus_create or Xilinx
      | concat block.
      | The input will be divided into the specified number
      | of outputs with the specified arithmetic types.
      | Divisions are made from most significant bit.
      mask init: same as sdbe_11_11/get_data_from_pkt/scope/bus_expand1
      settings: AttributesFormatString=8 outputs
      mask TypeOptions mode: divisions of equal size | divisions of arbitrary size
      mask Callback mode: bus_expand_callback();
      mask Callback outputWidth: bus_expand_callback();
      mask Callback outputToWorkspace: bus_expand_callback();
  bus_expand3 : Subsystem  AncestorBlock=casper_library_flow_control/bus_expand  mask(bus_expand){mode=divisions of equal size, outputNum=8, outputWidth=2, outputBinaryPt=0, outputArithmeticType=0, show_format=off, outputToWorkspace=off, variablePrefix=out, outputToModelAsWell=on}
      mask prompts: outputNum "Number of outputs:"; outputWidth "Output width:"; outputBinaryPt "Output binary point position:"; outputArithmeticType "Output arithmetic type (ufix=0, fix=1, bool=2):"; show_format "Print format string?"; outputToWorkspace "Output to workspace?"; variablePrefix "Variable name prefix:"; outputToModelAsWell "Output to model as well?"
      mask help:
      | Expands a 'bus' made using a bus_create or Xilinx
      | concat block.
      | The input will be divided into the specified number
      | of outputs with the specified arithmetic types.
      | Divisions are made from most significant bit.
      mask init: same as sdbe_11_11/get_data_from_pkt/scope/bus_expand1
      settings: AttributesFormatString=8 outputs
      mask TypeOptions mode: divisions of equal size | divisions of arbitrary size
      mask Callback mode: bus_expand_callback();
      mask Callback outputWidth: bus_expand_callback();
      mask Callback outputToWorkspace: bus_expand_callback();
  wires:
  val/1 -> Gateway Out34/1, Gateway Out24/1, Gateway Out14/1, Gateway Out3/1
  Constant/1 -> Mux/2
  [val_45] -> Mux/1
  Mux1/1 -> Scope/2  "val_yellow__w45_val_pink"
  Gateway Out3/1 -> Mux1/1
  Gateway Out4/1 -> Mux1/2
  data/1 -> Mux/3
  spec_val/1 -> Gateway Out35/1, Gateway Out25/1, Gateway Out15/1, Gateway Out4/1, [val_45]
  Gateway Out2/1 -> Mux2/2  "ref_ep_yellow________frame_num_pink"
  Gateway Out1/1 -> Mux2/1
  Gateway Out5/1 -> Mux2/3
  Gateway Out6/1 -> Mux2/4
  Mux2/1 -> Scope/1  "p0r"
  Mux/1 -> Subsystem/1(In5)
  Subsystem/1(p0r) -> [p0r]
  Subsystem/3(p1r) -> [p1r]
  Subsystem/4(p1i) -> [p1i]
  Subsystem/2(p0i) -> [p0i]
  Gateway Out8/1 -> Mux2/6  "ref_ep_yellow________frame_num_pink"
  Gateway Out7/1 -> Mux2/5
  Gateway Out9/1 -> Mux2/7
  Gateway Out10/1 -> Mux2/8
  bus_expand/1(msb_out8) -> Gateway Out1/1
  bus_expand/2(out7) -> Gateway Out2/1
  bus_expand/3(out6) -> Gateway Out5/1
  bus_expand/4(out5) -> Gateway Out6/1
  bus_expand/5(out4) -> Gateway Out7/1
  bus_expand/6(out3) -> Gateway Out8/1
  bus_expand/7(out2) -> Gateway Out9/1
  bus_expand/8(lsb_out1) -> Gateway Out10/1
  [p0r] -> bus_expand/1(bus_in)
  Mux3/1 -> Scope1/2  "val_yellow__w45_val_pink"
  Gateway Out14/1 -> Mux3/1
  Gateway Out15/1 -> Mux3/2
  Gateway Out13/1 -> Mux4/2  "ref_ep_yellow________frame_num_pink"
  Gateway Out11/1 -> Mux4/1
  Gateway Out16/1 -> Mux4/3
  Gateway Out17/1 -> Mux4/4
  Mux4/1 -> Scope1/1  "p0i"
  Gateway Out19/1 -> Mux4/6  "ref_ep_yellow________frame_num_pink"
  Gateway Out18/1 -> Mux4/5
  Gateway Out20/1 -> Mux4/7
  Gateway Out12/1 -> Mux4/8
  bus_expand1/1(msb_out8) -> Gateway Out11/1
  bus_expand1/2(out7) -> Gateway Out13/1
  bus_expand1/3(out6) -> Gateway Out16/1
  bus_expand1/4(out5) -> Gateway Out17/1
  bus_expand1/5(out4) -> Gateway Out18/1
  bus_expand1/6(out3) -> Gateway Out19/1
  bus_expand1/7(out2) -> Gateway Out20/1
  bus_expand1/8(lsb_out1) -> Gateway Out12/1
  [p0i] -> bus_expand1/1(bus_in)
  Mux5/1 -> Scope2/2  "val_yellow__w45_val_pink"
  Gateway Out24/1 -> Mux5/1
  Gateway Out25/1 -> Mux5/2
  Gateway Out23/1 -> Mux6/2  "ref_ep_yellow________frame_num_pink"
  Gateway Out21/1 -> Mux6/1
  Gateway Out26/1 -> Mux6/3
  Gateway Out27/1 -> Mux6/4
  Mux6/1 -> Scope2/1  "p1r"
  Gateway Out29/1 -> Mux6/6  "ref_ep_yellow________frame_num_pink"
  Gateway Out28/1 -> Mux6/5
  Gateway Out30/1 -> Mux6/7
  Gateway Out22/1 -> Mux6/8
  bus_expand2/1(msb_out8) -> Gateway Out21/1
  bus_expand2/2(out7) -> Gateway Out23/1
  bus_expand2/3(out6) -> Gateway Out26/1
  bus_expand2/4(out5) -> Gateway Out27/1
  bus_expand2/5(out4) -> Gateway Out28/1
  bus_expand2/6(out3) -> Gateway Out29/1
  bus_expand2/7(out2) -> Gateway Out30/1
  bus_expand2/8(lsb_out1) -> Gateway Out22/1
  [p0i] -> bus_expand2/1(bus_in)
  Mux7/1 -> Scope3/2  "val_yellow__w45_val_pink"
  Gateway Out34/1 -> Mux7/1
  Gateway Out35/1 -> Mux7/2
  Gateway Out33/1 -> Mux8/2  "ref_ep_yellow________frame_num_pink"
  Gateway Out31/1 -> Mux8/1
  Gateway Out36/1 -> Mux8/3
  Gateway Out37/1 -> Mux8/4
  Mux8/1 -> Scope3/1  "p1i"
  Gateway Out39/1 -> Mux8/6  "ref_ep_yellow________frame_num_pink"
  Gateway Out38/1 -> Mux8/5
  Gateway Out40/1 -> Mux8/7
  Gateway Out32/1 -> Mux8/8
  bus_expand3/1(msb_out8) -> Gateway Out31/1
  bus_expand3/2(out7) -> Gateway Out33/1
  bus_expand3/3(out6) -> Gateway Out36/1
  bus_expand3/4(out5) -> Gateway Out37/1
  bus_expand3/5(out4) -> Gateway Out38/1
  bus_expand3/6(out3) -> Gateway Out39/1
  bus_expand3/7(out2) -> Gateway Out40/1
  bus_expand3/8(lsb_out1) -> Gateway Out32/1
  [p0i] -> bus_expand3/1(bus_in)

== system sdbe_11_11/vdif_2/hdr_to_scope3/vtp ==
  note: VTP so need to wait one more clock
  data : Inport
  val : Inport  Port=2
  spec_val : Inport  Port=3
  Constant : xbsIndex_r4/Constant  const=0  gui_display_data_type=Fixed-point  arith_type=Unsigned  n_bits=64  bin_pt=0  preci_type=Single  exp_width=8  frac_width=24  explicit_period=on  period=1  equ=P=C  opselect=C  inp2=PCIN>>17  opr=+  inp1=P  carry=CIN  dbl_ovrd=off  block_type=constant
  Disregard Subsystem : xbsIndex_r4/Disregard Subsystem  Tag=discardX  block_type=disregard
  Gateway Out2 : xbsIndex_r4/Gateway Out  inherit_from_input=off  hdl_port=on  timing_constraint=None  locs_specified=off  LOCs={}  UseAsDAC=off  DACChannel='1'  block_type=gatewayout
  Gateway Out3 : xbsIndex_r4/Gateway Out  inherit_from_input=off  hdl_port=on  timing_constraint=None  locs_specified=off  LOCs={}  UseAsDAC=off  DACChannel='1'  block_type=gatewayout
  Gateway Out4 : xbsIndex_r4/Gateway Out  inherit_from_input=off  hdl_port=on  timing_constraint=None  locs_specified=off  LOCs={}  UseAsDAC=off  DACChannel='1'  block_type=gatewayout
  Mux : xbsIndex_r4/Mux  inputs=2  en=off  latency=0  precision=Full  arith_type=Unsigned  n_bits=16  bin_pt=14  quantization=Truncate  overflow=Wrap  dbl_ovrd=off  block_type=mux
  Mux1 : Mux  Inputs=2
  Scope : Scope  NumInputPorts=2
      settings: TimeRange=1.649420126233963  YMin=-1~-1  YMax=1~1  SaveName=ScopeData12
  get_frame_and_ref_ep : Subsystem
  wires:
  val/1 -> Gateway Out3/1
  Constant/1 -> Mux/2
  Mux/1 -> get_frame_and_ref_ep/1(hdr_64)
  [val_45] -> Mux/1
  Mux1/1 -> Scope/2  "val_yellow__w45_val_pink"
  get_frame_and_ref_ep/1(Out1) -> Gateway Out2/1
  Gateway Out3/1 -> Mux1/1
  Gateway Out4/1 -> Mux1/2
  data/1 -> Mux/3
  spec_val/1 -> Gateway Out4/1, [val_45]
  Gateway Out2/1 -> Scope/1  "vtp_num"

== system sdbe_11_11/vdif_2/hdr_to_scope3/w01 ==
  note: VTP so need to wait one more clock
  data : Inport
  val : Inport  Port=2
  spec_val : Inport  Port=3
  Constant : xbsIndex_r4/Constant  const=0  gui_display_data_type=Fixed-point  arith_type=Unsigned  n_bits=64  bin_pt=0  preci_type=Single  exp_width=8  frac_width=24  explicit_period=on  period=1  equ=P=C  opselect=C  inp2=PCIN>>17  opr=+  inp1=P  carry=CIN  dbl_ovrd=off  block_type=constant
  Disregard Subsystem : xbsIndex_r4/Disregard Subsystem  Tag=discardX  block_type=disregard
  Gateway Out{2..8} (7 alike) : xbsIndex_r4/Gateway Out  inherit_from_input=off  hdl_port=on  timing_constraint=None  locs_specified=off  LOCs={}  UseAsDAC=off  DACChannel='1'  block_type=gatewayout
  Mux : xbsIndex_r4/Mux  inputs=2  en=off  latency=0  precision=Full  arith_type=Unsigned  n_bits=16  bin_pt=14  quantization=Truncate  overflow=Wrap  dbl_ovrd=off  block_type=mux
  Mux1 : Mux  Inputs=2
  Mux2 : Mux  Inputs=2
  Mux3 : Mux  Inputs=2
  Scope : Scope  NumInputPorts=2
      settings: TimeRange=1.649420126233963  YMin=-1~-1  YMax=1~1  SaveName=ScopeData13
  Scope1 : Scope  NumInputPorts=2
      settings: TimeRange=1.649420126233963  YMin=-1~-1  YMax=1~1  SaveName=ScopeData15
  bus_expand : Subsystem  AncestorBlock=casper_library_flow_control/bus_expand  mask(bus_expand){mode=divisions of equal size, outputNum=2, outputWidth=32, outputBinaryPt=0, outputArithmeticType=0, show_format=off, outputToWorkspace=off, variablePrefix=out, outputToModelAsWell=on}
      mask prompts: outputNum "Number of outputs:"; outputWidth "Output width:"; outputBinaryPt "Output binary point position:"; outputArithmeticType "Output arithmetic type (ufix=0, fix=1, bool=2):"; show_format "Print format string?"; outputToWorkspace "Output to workspace?"; variablePrefix "Variable name prefix:"; outputToModelAsWell "Output to model as well?"
      mask help:
      | Expands a 'bus' made using a bus_create or Xilinx
      | concat block.
      | The input will be divided into the specified number
      | of outputs with the specified arithmetic types.
      | Divisions are made from most significant bit.
      mask init: same as sdbe_11_11/get_data_from_pkt/scope/bus_expand1
      settings: AttributesFormatString=2 outputs
      mask TypeOptions mode: divisions of equal size | divisions of arbitrary size
      mask Callback mode: bus_expand_callback();
      mask Callback outputWidth: bus_expand_callback();
      mask Callback outputToWorkspace: bus_expand_callback();
  get_frame_and_ref_ep : Subsystem
  get_secs_from_data : Subsystem
  wires:
  Gateway Out2/1 -> Scope/1  "seconds_since_ep"
  spec_val/1 -> [val_45], Gateway Out4/1
  data/1 -> Mux/3
  Gateway Out4/1 -> Mux1/2
  Gateway Out3/1 -> Mux1/1
  get_secs_from_data/1(secs) -> Gateway Out2/1
  Mux1/1 -> Scope/2  "val_yellow__w45_val_pink"
  [val_45] -> Mux/1
  Mux/1 -> bus_expand/1(bus_in)
  Constant/1 -> Mux/2
  val/1 -> Gateway Out3/1, Gateway Out5/1
  [w1] -> get_frame_and_ref_ep/1(hdr_64)
  bus_expand/1(msb_out2) -> [w0]
  bus_expand/2(lsb_out1) -> [w1]
  [w0] -> get_secs_from_data/1(hdr_64)
  Mux2/1 -> Scope1/1  "ref_ep_yellow_____frame_num_pink"
  get_frame_and_ref_ep/1(ref_ep) -> Gateway Out7/1
  get_frame_and_ref_ep/2(frame_num) -> Gateway Out8/1
  Gateway Out6/1 -> Mux3/2
  Gateway Out5/1 -> Mux3/1
  Mux3/1 -> Scope1/2  "val_yellow__w45_val_pink"
  [val_45] -> Gateway Out6/1
  Gateway Out7/1 -> Mux2/1
  Gateway Out8/1 -> Mux2/2

== system sdbe_11_11/vdif_2/hdr_to_scope3/w23 ==
  note: VTP so need to wait one more clock
  data : Inport
  val : Inport  Port=2
  spec_val : Inport  Port=3
  Constant : xbsIndex_r4/Constant  const=0  gui_display_data_type=Fixed-point  arith_type=Unsigned  n_bits=64  bin_pt=0  preci_type=Single  exp_width=8  frac_width=24  explicit_period=on  period=1  equ=P=C  opselect=C  inp2=PCIN>>17  opr=+  inp1=P  carry=CIN  dbl_ovrd=off  block_type=constant
  Disregard Subsystem : xbsIndex_r4/Disregard Subsystem  Tag=discardX  block_type=disregard
  Gateway Out{1..6} (6 alike) : xbsIndex_r4/Gateway Out  inherit_from_input=off  hdl_port=on  timing_constraint=None  locs_specified=off  LOCs={}  UseAsDAC=off  DACChannel='1'  block_type=gatewayout
  Mux : xbsIndex_r4/Mux  inputs=2  en=off  latency=0  precision=Full  arith_type=Unsigned  n_bits=16  bin_pt=14  quantization=Truncate  overflow=Wrap  dbl_ovrd=off  block_type=mux
  Mux1 : Mux  Inputs=2
  Mux2 : Mux  Inputs=2
  Scope : Scope  NumInputPorts=2
      settings: TimeRange=1.649420126233963  YMin=-1~-1  YMax=1~1  SaveName=ScopeData12
  Scope1 : Scope  NumInputPorts=2
      settings: TimeRange=1.649420126233963  YMin=-1~-1  YMax=1~1  SaveName=ScopeData16
  Subsystem : Subsystem
  Subsystem1 : Subsystem
  bus_expand : Subsystem  AncestorBlock=casper_library_flow_control/bus_expand  mask(bus_expand){mode=divisions of equal size, outputNum=2, outputWidth=32, outputBinaryPt=0, outputArithmeticType=0, show_format=off, outputToWorkspace=off, variablePrefix=out, outputToModelAsWell=on}
      mask prompts: outputNum "Number of outputs:"; outputWidth "Output width:"; outputBinaryPt "Output binary point position:"; outputArithmeticType "Output arithmetic type (ufix=0, fix=1, bool=2):"; show_format "Print format string?"; outputToWorkspace "Output to workspace?"; variablePrefix "Variable name prefix:"; outputToModelAsWell "Output to model as well?"
      mask help:
      | Expands a 'bus' made using a bus_create or Xilinx
      | concat block.
      | The input will be divided into the specified number
      | of outputs with the specified arithmetic types.
      | Divisions are made from most significant bit.
      mask init: same as sdbe_11_11/get_data_from_pkt/scope/bus_expand1
      settings: AttributesFormatString=2 outputs
      mask TypeOptions mode: divisions of equal size | divisions of arbitrary size
      mask Callback mode: bus_expand_callback();
      mask Callback outputWidth: bus_expand_callback();
      mask Callback outputToWorkspace: bus_expand_callback();
  wires:
  spec_val/1 -> [val_45], Gateway Out4/1
  data/1 -> Mux/3
  Gateway Out4/1 -> Mux1/2
  Gateway Out3/1 -> Mux1/1
  Mux1/1 -> Scope/2  "val_yellow__w45_val_pink"
  [val_45] -> Mux/1
  Constant/1 -> Mux/2
  val/1 -> Gateway Out5/1, Gateway Out3/1
  Mux/1 -> bus_expand/1(bus_in)
  bus_expand/1(msb_out2) -> [w0]
  bus_expand/2(lsb_out1) -> [w1]
  [w0] -> Subsystem/1(w2)
  Subsystem/1(frame_len) -> Gateway Out1/1
  Gateway Out1/1 -> Scope/1  "frame_len"
  Gateway Out6/1 -> Mux2/2
  Gateway Out5/1 -> Mux2/1
  Mux2/1 -> Scope1/2  "val_yellow__w45_val_pink"
  [w1] -> Subsystem1/1(w2)
  Subsystem1/1(stat_id) -> Gateway Out2/1
  Gateway Out2/1 -> Scope1/1
  [val_45] -> Gateway Out6/1
